simulink subsystem "s2s22e"  (R2022b)
settings: Solver=VariableStepAuto  StartTime=0.0  StopTime=10.0  RelTol=1e-3
settings Model: Creator=jack  LastModifiedBy=jack

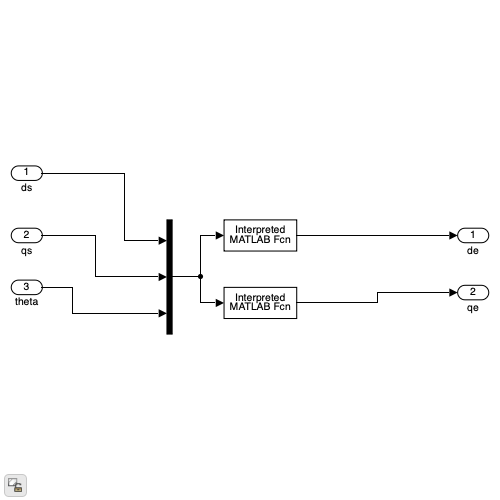
[thumbnail: Simulink's stored preview of the top-level diagram]
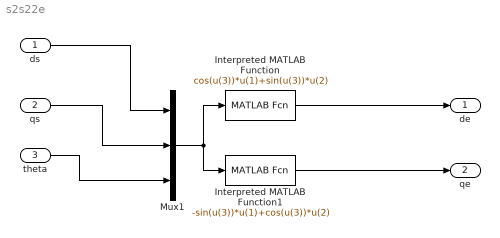
== system s2s22e ==
  ds : Inport
  qs : Inport  Port=2
  theta : Inport  Port=3
  Interpreted MATLAB Function : MATLABFcn  MATLABFcn=cos(u(3))*u(1)+sin(u(3))*u(2)
  Interpreted MATLAB Function1 : MATLABFcn  MATLABFcn=-sin(u(3))*u(1)+cos(u(3))*u(2)
  Mux1 : Mux  Inputs=3
  de : Outport
  qe : Outport  Port=2
  wires:
  Interpreted MATLAB Function1/1 -> qe/1
  qs/1 -> Mux1/2
  ds/1 -> Mux1/1
  Mux1/1 -> Interpreted MATLAB Function1/1, Interpreted MATLAB Function/1
  Interpreted MATLAB Function/1 -> de/1
  theta/1 -> Mux1/3
